simulink model "Part2"  (R2017a)
settings: Solver=VariableStepAuto  StartTime=0.0  StopTime=10.0  RelTol=1e-3
libraries: simulink x1
settings Model: Creator=RichardTorti  LastModifiedBy=RichardTorti

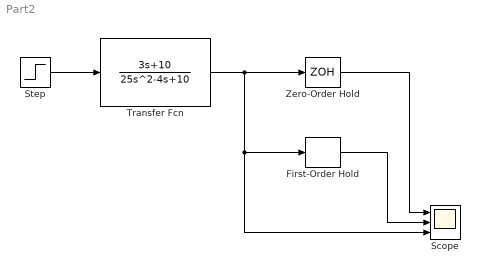
== system Part2 ==
  First-Order Hold : simulink/Discrete/First-Order Hold  DisableCoverage=on  Ts=0.3
      settings: SourceProductName=Simulink  SourceProductBaseCode=SL
  Scope : Scope  NumInputPorts=3
  Step : Step  Time=0  SampleTime=0
  Transfer Fcn : TransferFcn  Numerator=[3 10]  Denominator=[25 -4 10]
  Zero-Order Hold : ZeroOrderHold  SampleTime=0.3
  wires:
  Step/1 -> Transfer Fcn/1
  Transfer Fcn/1 -> Scope/3, First-Order Hold/1, Zero-Order Hold/1
  First-Order Hold/1 -> Scope/2
  Zero-Order Hold/1 -> Scope/1
